simulink model "robust_tracking"  (R2020b)
settings: Solver=VariableStepAuto  StartTime=0.0  StopTime=20.0  RelTol=1e-3
values from neighbouring files (symbols this model uses):
  drv =     [balrob_params.mat]
  g = 9.81    [balrob_params.mat]    (also in sfun_balrob_long_dyn.m)
  gbox =     [balrob_params.mat]    (also in sfun_balrob_long_dyn.m = block.DialogPrm(4).Data)
  ms22g = 0.101936799185    [balrob_params.mat]
  sens =     [balrob_params.mat]
  Ts = 0.01    [balrob_params.mat]
  wheel =     [balrob_params.mat]    (also in sfun_balrob_long_dyn.m = block.DialogPrm(5).Data)
undefined symbols (not defined in the file or in its folder): C_gain, denHw, denLPFz, DiscIntNeverNeededParam, Ki, N_u, N_x, numHw, numLPFz, step_disturbance, step_size, T
settings Model: Creator=39345  LastModifiedBy=Andrea
settings DataIOCC: ReturnWorkspaceOutputs=off

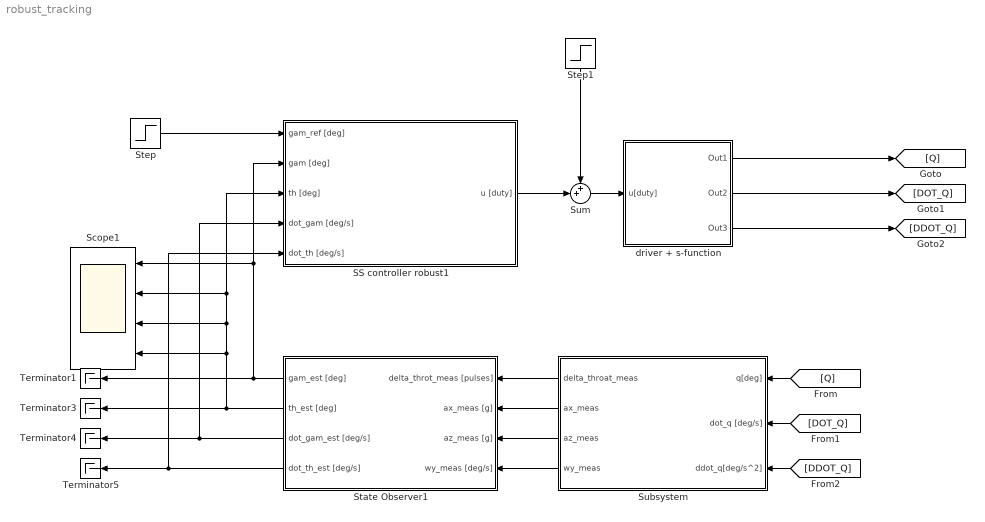
== system robust_tracking ==
  SS controller robust1 : Subsystem
  Scope1 : Scope  NumInputPorts=4
  State Observer1 : Subsystem
  Step : Step  After=step_size  SampleTime=0.01
  Step1 : Step  Time=11  After=step_disturbance  SampleTime=0.01
  Subsystem : Subsystem
  Sum : Sum  Inputs=++|
  Terminator{1,3..5} (4 alike) : Terminator
  driver + s-function : Subsystem
  wires:
  SS controller robust1/1(u [duty]) -> Sum/2
  Sum/1 -> driver + s-function/1(u[duty])
  Step/1 -> SS controller robust1/1(gam_ref [deg])
  Step1/1 -> Sum/1
  [DOT_Q] -> Subsystem/2(dot_q [deg/s])
  Subsystem/4(wy_meas) -> State Observer1/4(wy_meas [deg/s])
  [DDOT_Q] -> Subsystem/3(ddot_q[deg/s^2])
  Subsystem/3(az_meas) -> State Observer1/3("az_meas [g] ")
  [Q] -> Subsystem/1(q[deg])
  Subsystem/1(delta_throat_meas) -> State Observer1/1("delta_throt_meas [pulses] ")
  Subsystem/2(ax_meas) -> State Observer1/2("ax_meas [g] ")
  driver + s-function/2(Out2) -> [DOT_Q]
  driver + s-function/1(Out1) -> [Q]
  driver + s-function/3(Out3) -> [DDOT_Q]
  State Observer1/3(dot_gam_est [deg/s]) -> SS controller robust1/4(dot_gam [deg/s]), Terminator4/1
  State Observer1/4(dot_th_est [deg/s]) -> SS controller robust1/5(dot_th [deg/s]), Terminator5/1
  State Observer1/2(th_est [deg]) -> Scope1/2, SS controller robust1/3(th [deg]), Scope1/3, Scope1/4, Terminator3/1
  State Observer1/1(gam_est [deg]) -> Scope1/1, SS controller robust1/2(gam [deg]), Terminator1/1

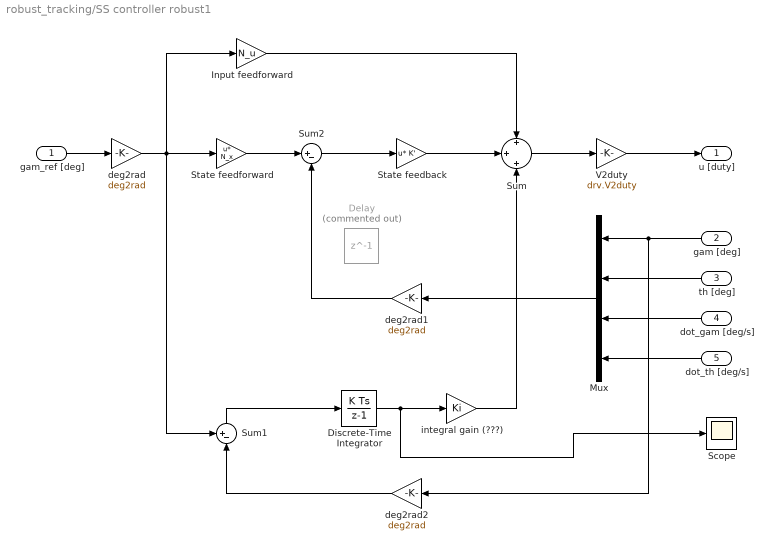
== system robust_tracking/SS controller robust1 ==
  gam_ref [deg] : Inport
  gam [deg] : Inport  Port=2
  th [deg] : Inport  Port=3
  dot_gam [deg/s] : Inport  Port=4
  dot_th [deg/s] : Inport  Port=5
  Delay : Delay  Commented=on  DelayLength=1  InitialCondition=0
  Discrete-Time Integrator : DiscreteIntegrator  SampleTime=0.01  ICPrevOutput=DiscIntNeverNeededParam  ICPrevScaledInput=DiscIntNeverNeededParam
  Input feedforward : Gain  Gain=N_u
  Mux : Mux
  Scope : Scope
  State feedback : Gain  Gain=K'  Multiplication=Matrix(u*K)
  "State feedforward\t" : Gain  Gain=N_x  Multiplication=Matrix(u*K)
  Sum : Sum  Inputs=+|+|+
  Sum1 : Sum  Inputs=+-|
  Sum2 : Sum  Inputs=|+-
  V2duty : Gain  Gain=drv.V2duty
  deg2rad : Gain  Gain=deg2rad
  deg2rad1 : Gain  Gain=deg2rad
  deg2rad2 : Gain  Gain=deg2rad
  integral gain (???) : Gain  Gain=Ki
  u [duty] : Outport
  wires:
  gam_ref [deg]/1 -> deg2rad/1
  deg2rad/1 -> Sum1/1, "State feedforward\t"/1, Input feedforward/1
  State feedback/1 -> Sum/2
  "State feedforward\t"/1 -> Sum2/1
  Sum2/1 -> State feedback/1
  Input feedforward/1 -> Sum/1
  Sum/1 -> V2duty/1
  V2duty/1 -> u [duty]/1
  gam [deg]/1 -> deg2rad2/1, Mux/1
  Mux/1 -> deg2rad1/1
  dot_gam [deg/s]/1 -> Mux/3
  th [deg]/1 -> Mux/2
  dot_th [deg/s]/1 -> Mux/4
  deg2rad1/1 -> Sum2/2
  deg2rad2/1 -> Sum1/2
  Sum1/1 -> Discrete-Time Integrator/1
  Discrete-Time Integrator/1 -> Scope/1, integral gain (???)/1
  integral gain (???)/1 -> Sum/3

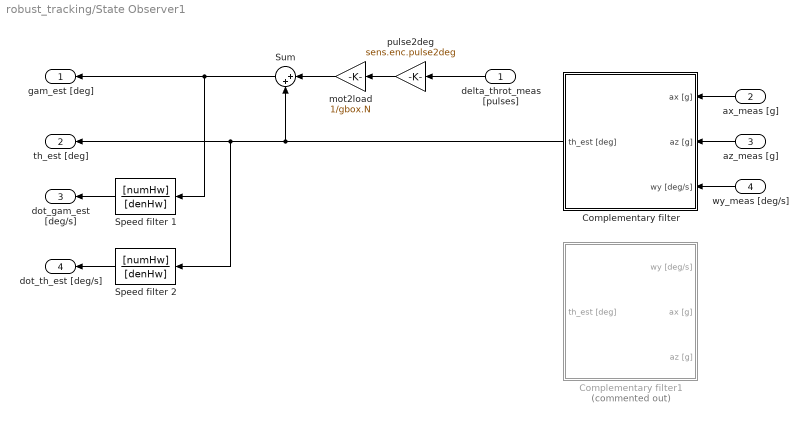
== system robust_tracking/State Observer1 ==
  "delta_throt_meas [pulses] " : Inport
  "ax_meas [g] " : Inport  Port=2
  "az_meas [g] " : Inport  Port=3
  wy_meas [deg/s] : Inport  Port=4
  Complementary filter : Subsystem
  Complementary filter1 : Subsystem  Commented=on
  Speed filter 1 : DiscreteTransferFcn  Numerator=[numHw]  Denominator=[denHw]  SampleTime=Ts
  Speed filter 2 : DiscreteTransferFcn  Numerator=[numHw]  Denominator=[denHw]  SampleTime=Ts
  Sum : Sum  Inputs=|++
  mot2load : Gain  Gain=1/gbox.N
  pulse2deg : Gain  Gain=sens.enc.pulse2deg
  gam_est [deg] : Outport
  th_est [deg] : Outport  Port=2
  dot_gam_est [deg/s] : Outport  Port=3
  dot_th_est [deg/s] : Outport  Port=4
  wires:
  pulse2deg/1 -> mot2load/1
  "delta_throt_meas [pulses] "/1 -> pulse2deg/1
  mot2load/1 -> Sum/1
  Complementary filter/1("th_est [deg] ") -> Sum/2, Speed filter 2/1, th_est [deg]/1
  Sum/1 -> Speed filter 1/1, gam_est [deg]/1
  Speed filter 1/1 -> dot_gam_est [deg/s]/1
  Speed filter 2/1 -> dot_th_est [deg/s]/1
  "ax_meas [g] "/1 -> Complementary filter/1("ax [g] ")
  "az_meas [g] "/1 -> Complementary filter/2("az [g] ")
  wy_meas [deg/s]/1 -> Complementary filter/3(wy [deg/s])

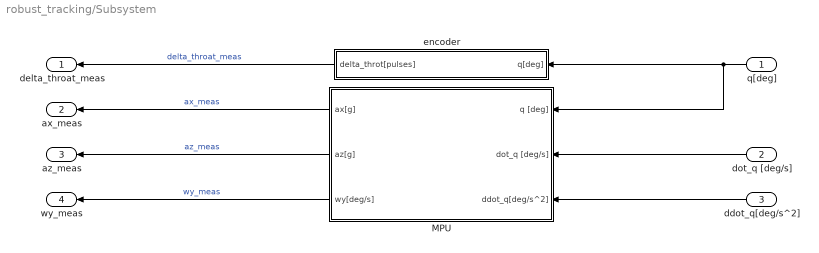
== system robust_tracking/Subsystem ==
  q[deg] : Inport
  dot_q [deg/s] : Inport  Port=2
  ddot_q[deg/s^2] : Inport  Port=3
  MPU : Subsystem
  encoder : Subsystem
  delta_throat_meas : Outport
  ax_meas : Outport  Port=2
  az_meas : Outport  Port=3
  wy_meas : Outport  Port=4
  wires:
  ddot_q[deg/s^2]/1 -> MPU/3(ddot_q[deg/s^2])
  q[deg]/1 -> MPU/1(q [deg]), encoder/1(q[deg])
  MPU/2(az[g]) -> az_meas/1  "az_meas"
  dot_q [deg/s]/1 -> MPU/2(dot_q [deg/s])
  encoder/1(delta_throt[pulses]) -> delta_throat_meas/1  "delta_throat_meas"
  MPU/1(ax[g]) -> ax_meas/1  "ax_meas"
  MPU/3(wy[deg/s]) -> wy_meas/1  "wy_meas"

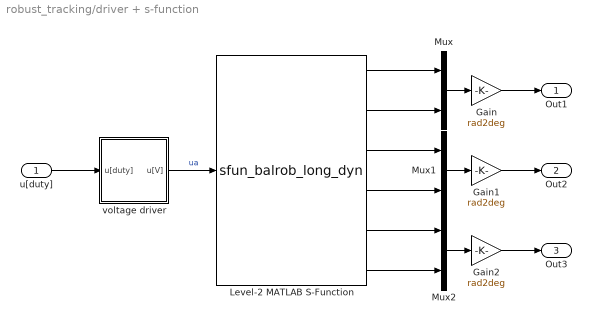
== system robust_tracking/driver + s-function ==
  u[duty] : Inport
  Gain : Gain  Gain=rad2deg
  Gain1 : Gain  Gain=rad2deg
  Gain2 : Gain  Gain=rad2deg
  "Level-2 MATLAB S-Function  " : M-S-Function  FunctionName=sfun_balrob_long_dyn  Parameters=x0, body, mot, gbox, wheel
  Mux : Mux  Inputs=2
  Mux1 : Mux  Inputs=2
  Mux2 : Mux  Inputs=2
  voltage driver : Subsystem
  Out1 : Outport
  Out2 : Outport  Port=2
  Out3 : Outport  Port=3
  wires:
  Mux/1 -> Gain/1
  "Level-2 MATLAB S-Function  "/3 -> Mux1/1
  "Level-2 MATLAB S-Function  "/2 -> Mux/2
  voltage driver/1(u[V]) -> "Level-2 MATLAB S-Function  "/1  "ua"
  Mux1/1 -> Gain1/1
  "Level-2 MATLAB S-Function  "/4 -> Mux1/2
  "Level-2 MATLAB S-Function  "/5 -> Mux2/1
  "Level-2 MATLAB S-Function  "/6 -> Mux2/2
  Gain2/1 -> Out3/1
  "Level-2 MATLAB S-Function  "/1 -> Mux/1
  Mux2/1 -> Gain2/1
  Gain1/1 -> Out2/1
  Gain/1 -> Out1/1
  u[duty]/1 -> voltage driver/1(u[duty])

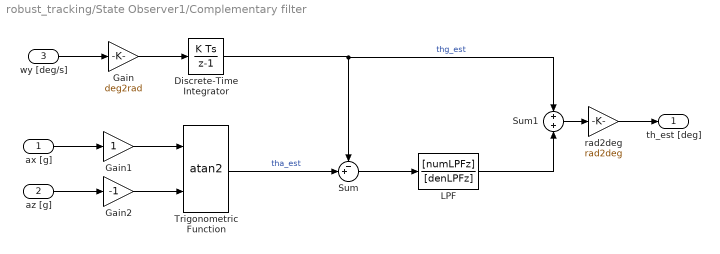
== system robust_tracking/State Observer1/Complementary filter ==
  "ax [g] " : Inport
  "az [g] " : Inport  Port=2
  wy [deg/s] : Inport  Port=3
  Discrete-Time Integrator : DiscreteIntegrator  gainval=1  SampleTime=Ts  ICPrevOutput=DiscIntNeverNeededParam  ICPrevScaledInput=DiscIntNeverNeededParam
  Gain : Gain  Gain=deg2rad
  Gain1 : Gain
  Gain2 : Gain  Gain=-1
  LPF : DiscreteTransferFcn  Numerator=[numLPFz]  Denominator=[denLPFz]  SampleTime=Ts
  Sum : Sum  Inputs=-+|
  Sum1 : Sum
  Trigonometric Function : Trigonometry  Operator=atan2
  rad2deg : Gain  Gain=rad2deg
  "th_est [deg] " : Outport
  wires:
  "az [g] "/1 -> Gain2/1
  "ax [g] "/1 -> Gain1/1
  wy [deg/s]/1 -> Gain/1
  Gain/1 -> Discrete-Time Integrator/1
  Gain2/1 -> Trigonometric Function/2
  Gain1/1 -> Trigonometric Function/1
  Trigonometric Function/1 -> Sum/2  "tha_est"
  Discrete-Time Integrator/1 -> Sum1/1, Sum/1  "thg_est"
  rad2deg/1 -> "th_est [deg] "/1
  Sum1/1 -> rad2deg/1
  Sum/1 -> LPF/1
  LPF/1 -> Sum1/2

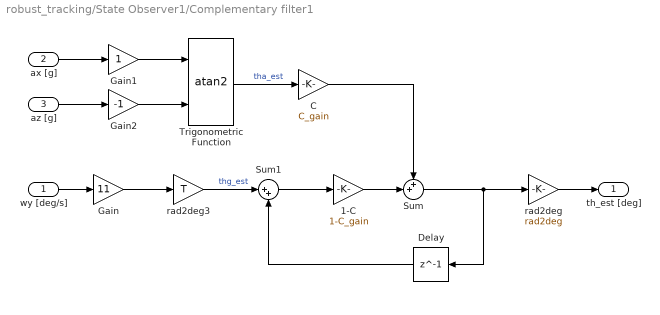
== system robust_tracking/State Observer1/Complementary filter1 ==
  wy [deg/s] : Inport
  "ax [g] " : Inport  Port=2
  "az [g] " : Inport  Port=3
  1-C : Gain  Gain=1-C_gain
  C : Gain  Gain=C_gain
  Delay : Delay  DelayLength=1
  Gain : Gain  Gain=11
  Gain1 : Gain
  Gain2 : Gain  Gain=-1
  Sum : Sum  Inputs=++|
  Sum1 : Sum  Inputs=|++
  Trigonometric Function : Trigonometry  Operator=atan2
  rad2deg : Gain  Gain=rad2deg
  rad2deg3 : Gain  Gain=T
  "th_est [deg] " : Outport
  wires:
  "az [g] "/1 -> Gain2/1
  "ax [g] "/1 -> Gain1/1
  wy [deg/s]/1 -> Gain/1
  Gain/1 -> rad2deg3/1
  Gain2/1 -> Trigonometric Function/2
  Gain1/1 -> Trigonometric Function/1
  rad2deg/1 -> "th_est [deg] "/1
  Trigonometric Function/1 -> C/1  "tha_est"
  C/1 -> Sum/1
  1-C/1 -> Sum/2
  Sum/1 -> Delay/1, rad2deg/1
  Delay/1 -> Sum1/2
  rad2deg3/1 -> Sum1/1  "thg_est"
  Sum1/1 -> 1-C/1

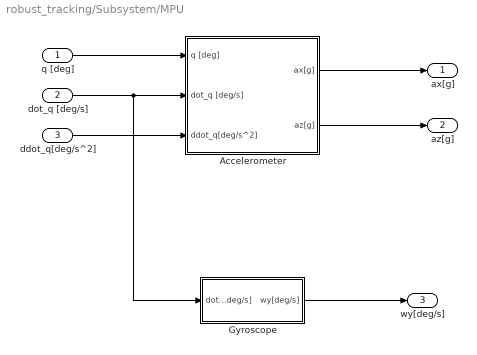
== system robust_tracking/Subsystem/MPU ==
  q [deg] : Inport
  dot_q [deg/s] : Inport  Port=2
  ddot_q[deg/s^2] : Inport  Port=3
  Accelerometer : Subsystem
  Gyroscope : Subsystem
  ax[g] : Outport
  az[g] : Outport  Port=2
  wy[deg/s] : Outport  Port=3
  wires:
  q [deg]/1 -> Accelerometer/1(q [deg])
  dot_q [deg/s]/1 -> Gyroscope/1(dot_q [deg/s]), Accelerometer/2(dot_q [deg/s])
  ddot_q[deg/s^2]/1 -> Accelerometer/3(ddot_q[deg/s^2])
  Gyroscope/1(wy[deg/s]) -> wy[deg/s]/1
  Accelerometer/1(ax[g]) -> ax[g]/1
  Accelerometer/2(az[g]) -> az[g]/1

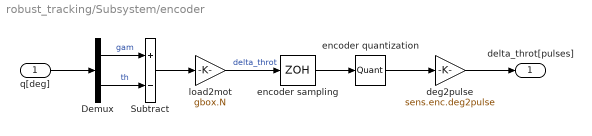
== system robust_tracking/Subsystem/encoder ==
  q[deg] : Inport
  Demux : Demux  Outputs=2
  Subtract : Sum  Inputs=+-
  deg2pulse : Gain  Gain=sens.enc.deg2pulse
  encoder quantization : Quantizer  QuantizationInterval=sens.enc.pulse2deg
  encoder sampling : ZeroOrderHold  SampleTime=Ts
  load2mot : Gain  Gain=gbox.N
  delta_throt[pulses] : Outport
  wires:
  q[deg]/1 -> Demux/1
  Demux/1 -> Subtract/1  "gam"
  Demux/2 -> Subtract/2  "th"
  Subtract/1 -> load2mot/1
  load2mot/1 -> encoder sampling/1  "delta_throt"
  encoder sampling/1 -> encoder quantization/1
  encoder quantization/1 -> deg2pulse/1
  deg2pulse/1 -> delta_throt[pulses]/1

== system robust_tracking/driver + s-function/voltage driver ==
  u[duty] : Inport
  Rounding Function : Rounding  Operator=fix
  Zero-Order Hold : ZeroOrderHold  SampleTime=Ts
  duty saturation : Saturate  UpperLimit=drv.dutymax  LowerLimit=-drv.dutymax
  duty2V : Gain  Gain=drv.duty2V
  voltage saturation1 : Saturate  UpperLimit=drv.Vbus  LowerLimit=-drv.Vbus
  u[V] : Outport
  wires:
  u[duty]/1 -> duty saturation/1
  duty saturation/1 -> Rounding Function/1
  Rounding Function/1 -> duty2V/1
  duty2V/1 -> voltage saturation1/1
  voltage saturation1/1 -> Zero-Order Hold/1
  Zero-Order Hold/1 -> u[V]/1

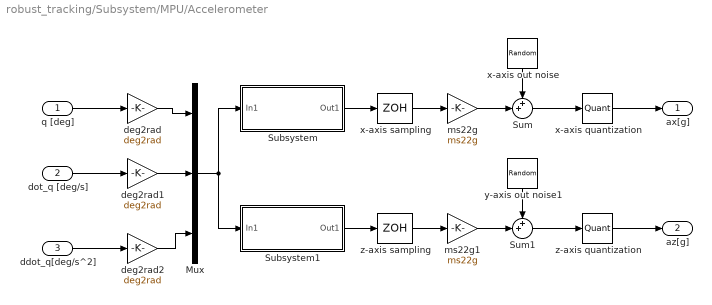
== system robust_tracking/Subsystem/MPU/Accelerometer ==
  q [deg] : Inport
  dot_q [deg/s] : Inport  Port=2
  ddot_q[deg/s^2] : Inport  Port=3
  Mux : Mux  Inputs=3
  Subsystem : Subsystem
  Subsystem1 : Subsystem
  Sum : Sum  Inputs=++|
  Sum1 : Sum  Inputs=++|
  deg2rad : Gain  Gain=deg2rad
  deg2rad1 : Gain  Gain=deg2rad
  deg2rad2 : Gain  Gain=deg2rad
  ms22g : Gain  Gain=ms22g
  ms22g1 : Gain  Gain=ms22g
  x-axis out noise : RandomNumber  Variance=sens.mpu.acc.noisevar  SampleTime=Ts
  x-axis quantization : Quantizer  QuantizationInterval=sens.mpu.acc.LSB2g
  x-axis sampling : ZeroOrderHold  SampleTime=Ts
  y-axis out noise1 : RandomNumber  Variance=sens.mpu.acc.noisevar  SampleTime=Ts
  z-axis quantization : Quantizer  QuantizationInterval=sens.mpu.acc.LSB2g
  z-axis sampling : ZeroOrderHold  SampleTime=Ts
  ax[g] : Outport
  az[g] : Outport  Port=2
  wires:
  ddot_q[deg/s^2]/1 -> deg2rad2/1
  dot_q [deg/s]/1 -> deg2rad1/1
  q [deg]/1 -> deg2rad/1
  deg2rad2/1 -> Mux/3
  deg2rad1/1 -> Mux/2
  deg2rad/1 -> Mux/1
  x-axis sampling/1 -> ms22g/1
  z-axis sampling/1 -> ms22g1/1
  x-axis out noise/1 -> Sum/1
  ms22g/1 -> Sum/2
  y-axis out noise1/1 -> Sum1/1
  ms22g1/1 -> Sum1/2
  Sum/1 -> x-axis quantization/1
  Sum1/1 -> z-axis quantization/1
  z-axis quantization/1 -> az[g]/1
  x-axis quantization/1 -> ax[g]/1
  Mux/1 -> Subsystem1/1(In1), Subsystem/1(In1)
  Subsystem/1(Out1) -> x-axis sampling/1
  Subsystem1/1(Out1) -> z-axis sampling/1

== system robust_tracking/Subsystem/MPU/Gyroscope ==
  dot_q [deg/s] : Inport
  Random Number : RandomNumber  Variance=sens.mpu.gyro.noisevar  SampleTime=Ts
  Selector2 : Selector  InputPortWidth=2  IndexOptions=Index vector (dialog)  Indices=2  OutputSizes=1
  Sum : Sum  Inputs=++|
  y-axis quantization : Quantizer  QuantizationInterval=sens.mpu.gyro.LSB2degs
  y-axis sampling : ZeroOrderHold  SampleTime=Ts
  wy[deg/s] : Outport
  wires:
  dot_q [deg/s]/1 -> Selector2/1
  Selector2/1 -> y-axis sampling/1
  y-axis sampling/1 -> Sum/2
  Random Number/1 -> Sum/1
  Sum/1 -> y-axis quantization/1
  y-axis quantization/1 -> wy[deg/s]/1

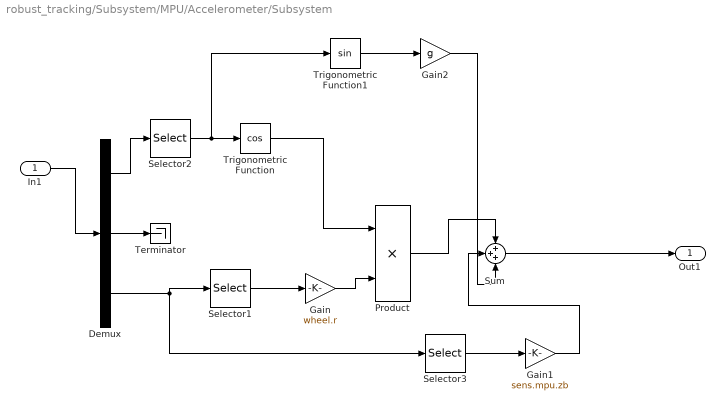
== system robust_tracking/Subsystem/MPU/Accelerometer/Subsystem ==
  In1 : Inport
  Demux : Demux  Outputs=3
  Gain : Gain  Gain=wheel.r
  Gain1 : Gain  Gain=sens.mpu.zb
  Gain2 : Gain  Gain=g
  Product : Product
  Selector1 : Selector  InputPortWidth=2  IndexOptions=Index vector (dialog)  Indices=1  OutputSizes=1
  Selector2 : Selector  InputPortWidth=2  IndexOptions=Index vector (dialog)  Indices=2  OutputSizes=1
  Selector3 : Selector  InputPortWidth=2  IndexOptions=Index vector (dialog)  Indices=2  OutputSizes=1
  Sum : Sum  Inputs=+++
  Terminator : Terminator
  Trigonometric Function : Trigonometry  Operator=cos
  Trigonometric Function1 : Trigonometry
  Out1 : Outport
  wires:
  In1/1 -> Demux/1
  Demux/3 -> Selector3/1, Selector1/1
  Selector1/1 -> Gain/1
  Demux/1 -> Selector2/1
  Selector2/1 -> Trigonometric Function1/1, Trigonometric Function/1
  Gain/1 -> Product/2
  Trigonometric Function/1 -> Product/1
  Product/1 -> Sum/1
  Sum/1 -> Out1/1
  Selector3/1 -> Gain1/1
  Trigonometric Function1/1 -> Gain2/1
  Gain1/1 -> Sum/2
  Gain2/1 -> Sum/3
  Demux/2 -> Terminator/1

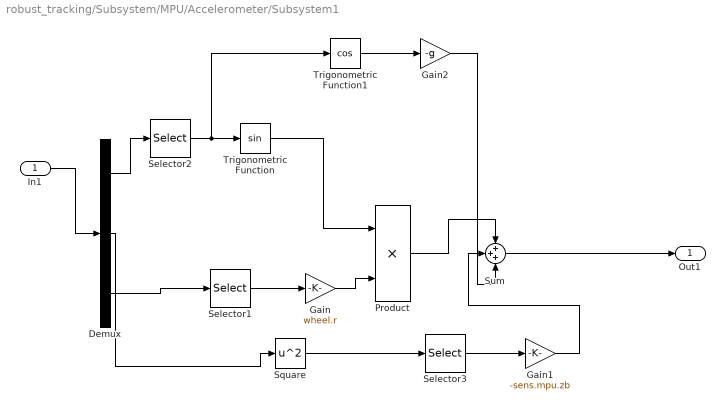
== system robust_tracking/Subsystem/MPU/Accelerometer/Subsystem1 ==
  In1 : Inport
  Demux : Demux  Outputs=3
  Gain : Gain  Gain=wheel.r
  Gain1 : Gain  Gain=-sens.mpu.zb
  Gain2 : Gain  Gain=-g
  Product : Product
  Selector1 : Selector  InputPortWidth=2  IndexOptions=Index vector (dialog)  Indices=1  OutputSizes=1
  Selector2 : Selector  InputPortWidth=2  IndexOptions=Index vector (dialog)  Indices=2  OutputSizes=1
  Selector3 : Selector  InputPortWidth=2  IndexOptions=Index vector (dialog)  Indices=2  OutputSizes=1
  Square : Math  Operator=square  SaturateOnIntegerOverflow=on
  Sum : Sum  Inputs=+++
  Trigonometric Function : Trigonometry
  Trigonometric Function1 : Trigonometry  Operator=cos
  Out1 : Outport
  wires:
  Selector1/1 -> Gain/1
  In1/1 -> Demux/1
  Demux/1 -> Selector2/1
  Selector3/1 -> Gain1/1
  Gain2/1 -> Sum/3
  Gain/1 -> Product/2
  Gain1/1 -> Sum/2
  Selector2/1 -> Trigonometric Function1/1, Trigonometric Function/1
  Trigonometric Function1/1 -> Gain2/1
  Trigonometric Function/1 -> Product/1
  Sum/1 -> Out1/1
  Product/1 -> Sum/1
  Demux/3 -> Selector1/1
  Demux/2 -> Square/1
  Square/1 -> Selector3/1
